simulink model "capitol8prob3"  (R2013a)
settings: Solver=ode45  StartTime=0.0  StopTime=2400  RelTol=1e-3
undefined symbols (not defined in the file): des, gcbh
settings Model: Creator=user  LastModifiedBy=user

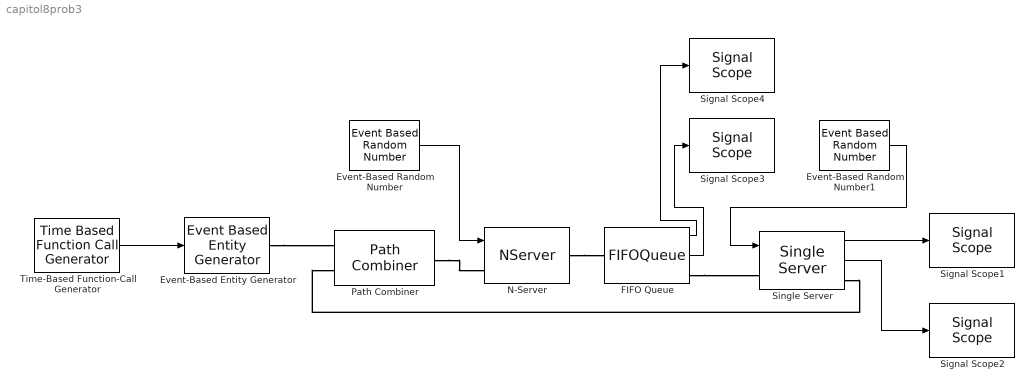
== system capitol8prob3 ==
  Event-Based Entity Generator : EventBasedEntityGenerator  GenerateEntitiesUpon=Function call from port fcn
  Event-Based Random Number : EventBasedRandomNumber  Distribution=Uniform  minUnif=25  maxUnif=35
  Event-Based Random Number1 : EventBasedRandomNumber  Distribution=Uniform  minUnif=6  maxUnif=10
  FIFO Queue : FIFOQueue  StatAverageWait=on  StatAverageQueueLength=on
      settings: OutputPortMap=o2,o3
  N-Server : NServer  NumberOfServers=4  ServiceTimeFrom=Signal port t
  Path Combiner : PathCombiner  NumberInputPorts=2
  Signal Scope{1..4} (4 alike) : SignalScope  LoadFcn=des.scope.CallbackSupport('seLoadFcn',gcbh)  StartFcn=des.scope.CallbackSupport('seStartFcn',gcbh)  StopFcn=des.scope.CallbackSupport('seStopFcn',gcbh)
      settings: CopyFcn=des.scope.CallbackSupport('seCopyFcn',gcbh)  DeleteFcn=des.scope.CallbackSupport('seDeleteFcn',gcbh)  PreSaveFcn=des.scope.CallbackSupport('sePreSaveFcn',gcbh)  NameChangeFcn=des.scope.CallbackSupport('seNameChangeFcn',gcbh)  OpenFcn=des.scope.CallbackSupport('seOpenFcn',gcbh)
  Single Server : SingleServer  ServiceTimeFrom=Signal port t  StatAverageWait=on  StatUtilization=on
      settings: OutputPortMap=o4,o5
  Time-Based Function-Call Generator : TimeBasedFunctionCallGenerator  NumberOfEventsPerPeriod=4
  wires:
  Time-Based Function-Call Generator/1 -> Event-Based Entity Generator/1
  Event-Based Random Number/1 -> N-Server/1
  Event-Based Random Number1/1 -> Single Server/1
  Single Server/2 -> Signal Scope2/1
  Single Server/1 -> Signal Scope1/1
  FIFO Queue/2 -> Signal Scope3/1
  FIFO Queue/1 -> Signal Scope4/1
  connections:
  Single Server/RConn1 -- Path Combiner/LConn2
  Event-Based Entity Generator/RConn1 -- Path Combiner/LConn1
  FIFO Queue/RConn1 -- Single Server/LConn1
  N-Server/RConn1 -- FIFO Queue/LConn1
  Path Combiner/RConn1 -- N-Server/LConn1
